simulink model "simulink_10_04_procede"  (R2024a)
settings: Solver=VariableStepAuto  StartTime=0.0  StopTime=600  RelTol=1e-3
StartFcn:
  | out = [];
  | disp(Consigne)
  |             disp(T_init);
  |             if Consigne > T_init
  |                 if T_init < 23
  |                     K1 = 0.007628;
  |                     T1 = 0.01103;
  |                     K2 = 0.03405;
  |                     T2 = 0.03035;
  |                     K3 = 0.04391;
  |                     T3 = 0.04924;
  |                 else
  |                     K1 = 0.00881;
  |                     T1 = 0.01194;
  |                     K2 = 0.02418;
  |                     T2 = 0.02359;
  |                     K3 = 0.04385;
  |                     T3 = 0.04942;
  |                 end
  |             else
  |                 if T_init < 30
  |                     K1 = 0.00751;
  |                     T1 = 0.01415;
  |                     K2 = 0.02291;
  |                     T2 = 0.02201;
  |                     K3 = 0.3512;
  |                     T3 = 0.3473;
  |                 else
  |                     K1 = 0.01043;
  |                     T1 = 0.01371;
  |                     K2 = 0.02568;
  |                     T2 = 0.0256;
  |                     K3 = 0.03719;
  |                     T3 = 0.04271;
  |                 end
  |             end
  |             disp('K1');
  |             disp(K1);
StopFcn:
  | try
  |     enreg = get_param('simulink_08_04_procede/Boucle Fermée', 'Enregistrement');
  |     nom = get_param('simulink_08_04_procede/Boucle Fermée', 'Fichier');
  | 
  |     if strcmp(enreg, 'on')
  |         dossier = fileparts(get_param('simulink_08_04_procede', 'FileName'));
  | 
  |         t = out.tout;
  |         y = out.Fichier;
  | 
  |         n = min(length(t), length(y));
  |         t_cut = t(1:n);
  |         y_cut = y(1:n, :);
  | 
  |         T = table(t_cut, y_cut(:,1), 'VariableNames', {'temps', 'sortie'});
  |         writetable(T, fullfile(dossier, [nom '.csv']));
  |     end
  | catch e
  |     disp(['Erreur exportation: ' e.message]);
  | end
values from neighbouring files (symbols this model uses):
  Consigne = ws.get('Consigne')    [logique.m]    (also in variables_simulation.m = 30)
  t_pertub_1 = 30    [variables_simulation.m]
  t_pertub_2 = 30    [variables_simulation.m]
  t_pertub_3 = 30    [variables_simulation.m]
settings Model: Creator=sabri  LastModifiedBy=MADER143
settings DataIOCC: OutputSaveName=y3

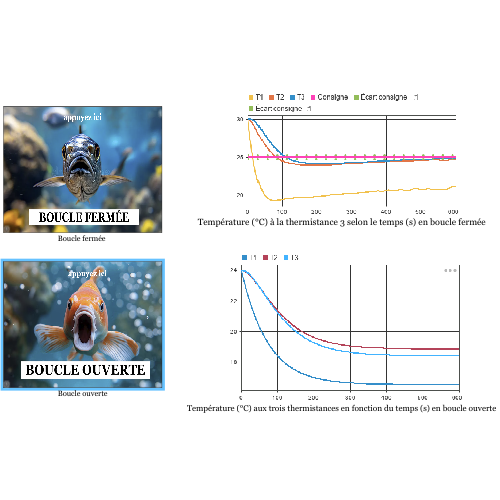
[thumbnail: Simulink's stored preview of the top-level diagram]
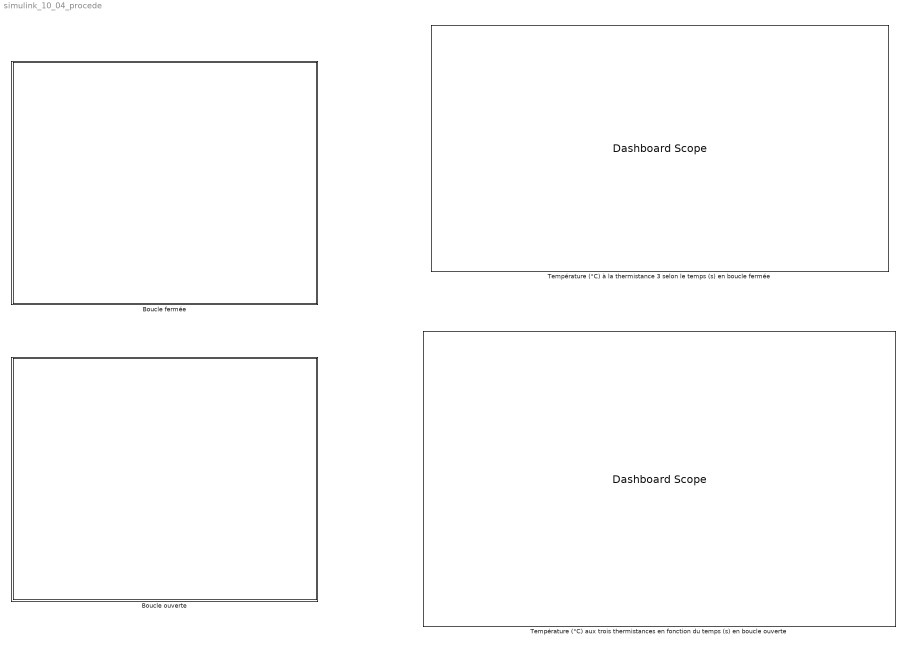
== system simulink_10_04_procede ==
  "Boucle fermée " : Subsystem  mask{Consigne=25, T_init=30, Temps=600, Enregistrement=on, Fichier=simulation, V1_3=1.79, Rg_3=5600, R1_3=3300, Rf_3=6300, B3=3700, V2_3=5, V1_2=1.8, Rg_2=5600, R1_2=3300, Rf_2=6300, B2=3984, V2_2=5, V1_1=1.774, Rg_1=5600, R1_1=3300, Rf_1=3300, B1=4010, V2_1=5, T_0=298.15, RT_0=10000, bz=-0.9726, az=0.0133, K1=0, T1=0, K2=0, T2=0, K3=0, T3=0, nb_bits=10, Ts=0.5, R=25, t_perturb_3=0, t_perturb_2=110, t_perturb_1=0, perturb_3=0, perturb_2=0.5, perturb_1=0, K=10.5, Ti=230, Td=40, PWM=0}
      mask prompts: Consigne "Température désirée"; T_init "Température initiale"; Temps "Durée de la simulation (s)"; Enregistrement "Enregistrer les données"; Fichier "Nom du fichier à enregistré:"; V1_3 "Tension d'alimentation de la branche positive de l'ampli-op (V)"; Rg_3 "Résistance en parallèle avec la thermitance (Ω)"; R1_3 "Résistance de la branche négative de l'ampli-op (Ω)"; Rf_3 "Résistance du trimpot (Ω)"; B3 "B"; V2_3 "Tension d'alimentation (V)"; V1_2 "Tension d'alimentation de la branche positive de l'ampli-op (V) de T1"; Rg_2 "Résistance en parallèle avec la thermitance (Ω)"; R1_2 "Résistance de la branche négative de l'ampli-op (Ω)"; Rf_2 "Résistance du trimpot (Ω)"; B2 "B"; V2_2 "Tension d'alimentation (V) de T1"; V1_1 "Tension d'alimentation de la branche positive de l'ampli-op (V) de T1"; Rg_1 "Résistance en parallèle avec la thermitance (Ω)"; R1_1 "Résistance de la branche négative de l'ampli-op (Ω)"; Rf_1 "Résistance du trimpot (Ω)"; B1 "B"; V2_1 "Tension d'alimentation (V) de T1"; T_0 "Température de référence de la thermistance (K)"; RT_0 "Résistance de référence de la thermistance (Ω)"; bz "Constante b"; az "Constante a"; K1 "Gain"; T1 "Constante de temps"; K2 "Gain"; T2 "Constante de temps"; K3 "Gain"; T3 "Constante de temps"; nb_bits "Nombre de bits du MC"; Ts "Fréquence d'échantillonnage"; R "Résistance de la perturbation (Ω)"; t_perturb_3 "Temps de la perturbation 3"; t_perturb_2 "Temps de la perturbation 2"; t_perturb_1 "Temps de la perturbation 1"; perturb_3 "Puissance de la perturbation à T3"; perturb_2 "Puissance de la perturbation à T2"; perturb_1 "Puissance de la perturbation à T1"; K "Gain"; Ti "Constante de temps intégrale"; Td "Constante de temps dérivée"
      mask DialogControl ParameterGroupVar Prompt: Simulateur
      mask DialogControl Container3 Prompt: Guide d'utilisation
      mask DialogControl Control2 Prompt: Voici le simulateur thermique de l'équipe 5. Vous pouvez modifier les valeurs des différents paramètres du prototype ci-dessus et choisir la température désirée.
      mask DialogControl Control3 Prompt: Lancer la simulation!
      mask DialogControl Container4 Prompt: Paramètres du prototype
      mask DialogControl Container8 Prompt: Paramètres des thermistances
      mask DialogControl Container9 Prompt: Thermistance 3
      mask DialogControl Container7 Prompt: Thermistance 2
      mask DialogControl Container5 Prompt: Thermistance 1
      mask DialogControl Container11 Prompt: Fonctions de transfert des thermistances
      mask DialogControl Container15 Prompt: T2 -> T3
      mask DialogControl Container12 Prompt: U -> V1
      mask DialogControl Container13 Prompt: V1 -> V2
      mask DialogControl Container14 Prompt: V2 -> V3
      mask DialogControl Container10 Prompt: Paramètres des perturbations
      mask DialogControl Container6 Prompt: Paramètres PID
      mask Display: image('boucle_fermee.png');
  Boucle ouverte : Subsystem  mask{PWM=-20, T_init=24, Temps=600, Enregistrement=on, Fichier=simulation, V1_3=1.79, Rg_3=5600, R1_3=3300, Rf_3=6300, B3=3700, V2_3=5, V1_2=1.8, Rg_2=5600, R1_2=3300, Rf_2=6300, B2=3984, V2_2=5, V1_1=1.774, Rg_1=5600, R1_1=3300, Rf_1=3300, B1=4010, V2_1=5, T_0=298.15, RT_0=10000, bz=-0.9726, az=0.0133, K1=0, T1=0, K2=0, T2=0, K3=0, T3=0, nb_bits=10, Ts=0.5, R=25, t_perturb_3=250, t_perturb_2=0, t_perturb_1=0, perturb_3=0, perturb_2=0, perturb_1=0, K=10.5, Ti=230, Td=40}
      mask prompts: PWM "PWM à envoyer"; T_init "Température initiale"; Temps "Durée de la simulation (s)"; Enregistrement "Enregistrer les données"; Fichier "Nom du fichier à enregistré:"; V1_3 "Tension d'alimentation de la branche positive de l'ampli-op (V)"; Rg_3 "Résistance en parallèle avec la thermitance (Ω)"; R1_3 "Résistance de la branche négative de l'ampli-op (Ω)"; Rf_3 "Résistance du trimpot (Ω)"; B3 "B"; V2_3 "Tension d'alimentation (V)"; V1_2 "Tension d'alimentation de la branche positive de l'ampli-op (V) de T1"; Rg_2 "Résistance en parallèle avec la thermitance (Ω)"; R1_2 "Résistance de la branche négative de l'ampli-op (Ω)"; Rf_2 "Résistance du trimpot (Ω)"; B2 "B"; V2_2 "Tension d'alimentation (V) de T1"; V1_1 "Tension d'alimentation de la branche positive de l'ampli-op (V) de T1"; Rg_1 "Résistance en parallèle avec la thermitance (Ω)"; R1_1 "Résistance de la branche négative de l'ampli-op (Ω)"; Rf_1 "Résistance du trimpot (Ω)"; B1 "B"; V2_1 "Tension d'alimentation (V) de T1"; T_0 "Température de référence de la thermistance (K)"; RT_0 "Résistance de référence de la thermistance (Ω)"; bz "Constante b"; az "Constante a"; K1 "Gain"; T1 "Constante de temps"; K2 "Gain"; T2 "Constante de temps"; K3 "Gain"; T3 "Constante de temps"; nb_bits "Nombre de bits du MC"; Ts "Fréquence d'échantillonnage"; R "Résistance de la perturbation (Ω)"; t_perturb_3 "Temps de la perturbation 3"; t_perturb_2 "Temps de la perturbation 2"; t_perturb_1 "Temps de la perturbation 1"; perturb_3 "Puissance de la perturbation à T3"; perturb_2 "Puissance de la perturbation à T2"; perturb_1 "Puissance de la perturbation à T1"; K "Gain"; Ti "Constante de temps intégrale"; Td "Constante de temps dérivée"
      mask DialogControl ParameterGroupVar Prompt: Simulateur
      mask DialogControl Container3 Prompt: Guide d'utilisation
      mask DialogControl Control2 Prompt: Voici le simulateur thermique en boucle ouverte de l'équipe 5. Vous pouvez modifier les valeurs des différents paramètres du prototype ci-dessus et choisir la consigne en PWM.
      mask DialogControl Control3 Prompt: Lancer la simulation!
      mask DialogControl Container4 Prompt: Paramètres du prototype
      mask DialogControl Container8 Prompt: Paramètres des thermistances
      mask DialogControl Container9 Prompt: Thermistance 3
      mask DialogControl Container7 Prompt: Thermistance 2
      mask DialogControl Container5 Prompt: Thermistance 1
      mask DialogControl Container11 Prompt: Fonctions de transfert des thermistances
      mask DialogControl Container15 Prompt: T2 -> T3
      mask DialogControl Container12 Prompt: U -> V1
      mask DialogControl Container13 Prompt: V1 -> V2
      mask DialogControl Container14 Prompt: V2 -> V3
      mask DialogControl Container10 Prompt: Paramètres des perturbations
      mask DialogControl Container6 Prompt: Paramètres PID
      mask Display: image('boucle_ouverte.png');
  Température (°C) aux trois thermistances en fonction du temps (s) en boucle ouverte : DashboardScope
  Température (°C) à la thermistance 3 selon le temps (s) en boucle fermée : DashboardScope

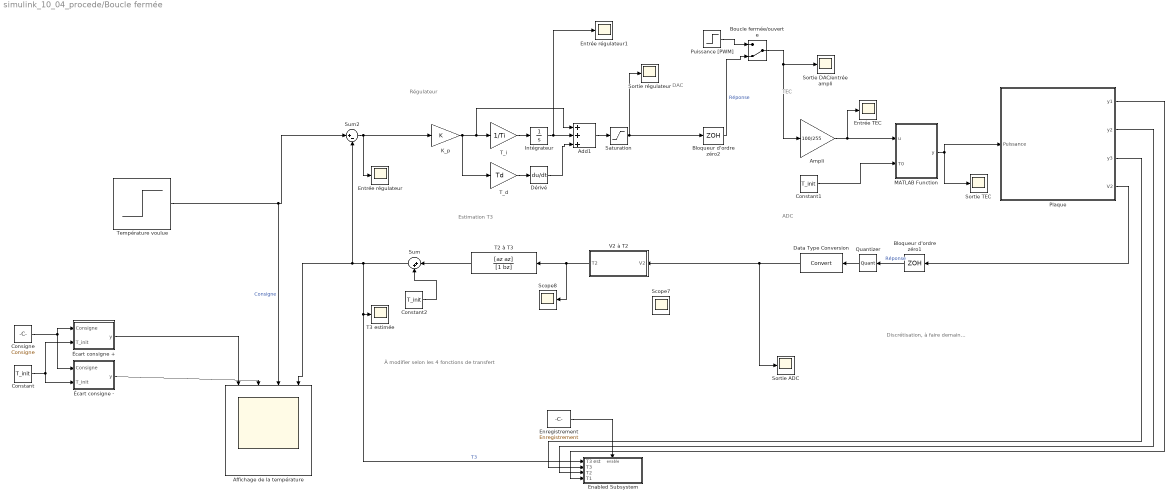
== system simulink_10_04_procede/Boucle fermée  ==
  note: À modifier selon les 4 fonctions de transfert
  note: Discrétisation, à faire demain...
  note: TEC
  note: DAC
  note: Régulateur
  note: Estimation T3
  note: ADC
  Add1 : Sum  Inputs=+++
  Affichage de la température : Scope  NumInputPorts=4
  Ampli : Gain  Gain=100/255
  Bloqueur d'ordre zéro1 : ZeroOrderHold  SampleTime=Ts
  Bloqueur d'ordre zéro2 : ZeroOrderHold  SampleTime=Ts
  Boucle fermée/ouverte : ManualSwitch  CurrentSetting=0
  Consigne : Constant  Value=Consigne
  Constant : Constant  Value=T_init
  Constant1 : Constant  Value=T_init
  Constant2 : Constant  Value=T_init
  Data Type Conversion : DataTypeConversion  OutMin=[-5]  OutMax=[5]  SaturateOnIntegerOverflow=off  RndMeth=Floor
  Dérivé : Derivative
  Enabled Subsystem : Subsystem  TreatAsAtomicUnit=on
  Enregistrement : Constant  Value=Enregistrement
  Entrée TEC : Scope
  Entrée régulateur : Scope
  Entrée régulateur1 : Scope
  Intégrateur : Integrator
  K_p : Gain  Gain=K
  MATLAB Function : MATLAB Function  TreatAsAtomicUnit=on
  Plaque : Subsystem
  Puissance [PWM] : Step  After=20  SampleTime=0
  Quantizer : Quantizer  QuantizationInterval=nb_bits/1023
  Saturation : Saturate  UpperLimit=70  LowerLimit=-70
  Scope7 : Scope
  Scope8 : Scope
  Sortie ADC : Scope
  Sortie DAC/entrée ampli : Scope
  Sortie TEC : Scope
  Sortie régulateur : Scope
  Sum : Sum  Inputs=|++
  Sum2 : Sum  Inputs=|+-
  T2 à T3 : DiscreteTransferFcn  Numerator=[az az]  Denominator=[1 bz]
  T3 estimée : Scope
  T_d : Gain  Gain=Td
  T_i : Gain  Gain=1/Ti
  Température voulue : Step  Time=0  Before=T_init  After=Consigne  SampleTime=0
  V2 à T2 : Subsystem
  Écart consigne + : MATLAB Function  TreatAsAtomicUnit=on
  Écart consigne - : MATLAB Function  TreatAsAtomicUnit=on
  wires:
  Écart consigne -/1(y) -> Affichage de la température/2
  Température voulue/1 -> Sum2/1, Affichage de la température/3  "Consigne"
  Écart consigne +/1(y) -> Affichage de la température/1
  Enregistrement/1 -> Enabled Subsystem/Enable
  Consigne/1 -> Écart consigne -/1(Consigne), Écart consigne +/1(Consigne)
  Constant/1 -> Écart consigne -/2(T_init), Écart consigne +/2(T_init)
  Boucle fermée/ouverte/1 -> Ampli/1, Sortie DAC/entrée ampli/1
  Intégrateur/1 -> Entrée régulateur1/1, Add1/2
  MATLAB Function/1(y) -> Plaque/1(Puissance), Sortie TEC/1
  Puissance [PWM]/1 -> Boucle fermée/ouverte/1
  Constant1/1 -> MATLAB Function/2(T0)
  Ampli/1 -> Entrée TEC/1, MATLAB Function/1(u)
  Sum2/1 -> Entrée régulateur/1, K_p/1
  T_i/1 -> Intégrateur/1
  Constant2/1 -> Sum/2
  V2 à T2/1(T2) -> T2 à T3/1, Scope8/1
  T2 à T3/1 -> Sum/1
  Add1/1 -> Saturation/1
  Saturation/1 -> Bloqueur d'ordre zéro2/1, Sortie régulateur/1
  Sum/1 -> Enabled Subsystem/1(T3 est), T3 estimée/1, Affichage de la température/4, Sum2/2  "T3"
  Quantizer/1 -> Data Type Conversion/1
  Plaque/4(V2) -> Bloqueur d'ordre zéro1/1
  Bloqueur d'ordre zéro1/1 -> Quantizer/1  "Réponse"
  Data Type Conversion/1 -> Sortie ADC/1, V2 à T2/1(V2)
  Bloqueur d'ordre zéro2/1 -> Boucle fermée/ouverte/2  "Réponse"
  K_p/1 -> T_d/1, Add1/1, T_i/1
  Dérivé/1 -> Add1/3
  T_d/1 -> Dérivé/1
  Plaque/2(y2) -> Enabled Subsystem/3(T2)
  Plaque/3(y3) -> Enabled Subsystem/2(T3)
  Plaque/1(y1) -> Enabled Subsystem/4(T1)

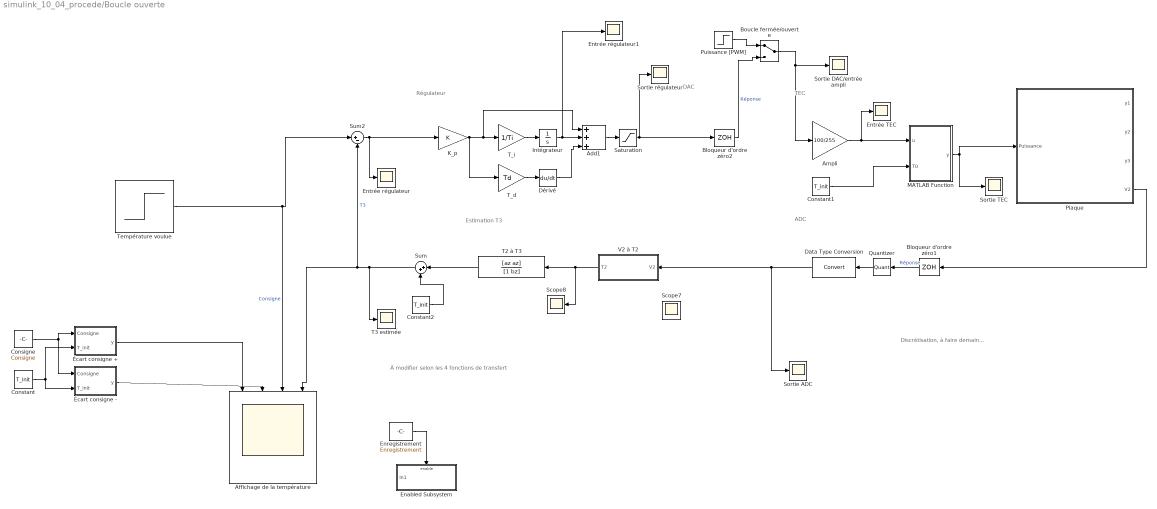
== system simulink_10_04_procede/Boucle ouverte ==
  note: À modifier selon les 4 fonctions de transfert
  note: Discrétisation, à faire demain...
  note: TEC
  note: DAC
  note: Régulateur
  note: Estimation T3
  note: ADC
  Add1 : Sum  Inputs=+++
  Affichage de la température : Scope  NumInputPorts=4
  Ampli : Gain  Gain=100/255
  Bloqueur d'ordre zéro1 : ZeroOrderHold  SampleTime=Ts
  Bloqueur d'ordre zéro2 : ZeroOrderHold  SampleTime=Ts
  Boucle fermée/ouverte : ManualSwitch
  Consigne : Constant  Value=Consigne
  Constant : Constant  Value=T_init
  Constant1 : Constant  Value=T_init
  Constant2 : Constant  Value=T_init
  Data Type Conversion : DataTypeConversion  OutMin=[-5]  OutMax=[5]  SaturateOnIntegerOverflow=off  RndMeth=Floor
  Dérivé : Derivative
  Enabled Subsystem : Subsystem  TreatAsAtomicUnit=on
  Enregistrement : Constant  Value=Enregistrement
  Entrée TEC : Scope
  Entrée régulateur : Scope
  Entrée régulateur1 : Scope
  Intégrateur : Integrator
  K_p : Gain  Gain=K
  MATLAB Function : MATLAB Function  TreatAsAtomicUnit=on
  Plaque : Subsystem
  Puissance [PWM] : Step  After=PWM  SampleTime=0
  Quantizer : Quantizer  QuantizationInterval=nb_bits/1023
  Saturation : Saturate  UpperLimit=70  LowerLimit=-70
  Scope7 : Scope
  Scope8 : Scope
  Sortie ADC : Scope
  Sortie DAC/entrée ampli : Scope
  Sortie TEC : Scope
  Sortie régulateur : Scope
  Sum : Sum  Inputs=|++
  Sum2 : Sum  Inputs=|+-
  T2 à T3 : DiscreteTransferFcn  Numerator=[az az]  Denominator=[1 bz]
  T3 estimée : Scope
  T_d : Gain  Gain=Td
  T_i : Gain  Gain=1/Ti
  Température voulue : Step  Time=0  Before=T_init  After=Consigne  SampleTime=0
  V2 à T2 : Subsystem
  Écart consigne + : MATLAB Function  TreatAsAtomicUnit=on
  Écart consigne - : MATLAB Function  TreatAsAtomicUnit=on
  wires:
  Écart consigne -/1(y) -> Affichage de la température/2
  Température voulue/1 -> Sum2/1, Affichage de la température/3  "Consigne"
  Écart consigne +/1(y) -> Affichage de la température/1
  Enregistrement/1 -> Enabled Subsystem/Enable
  Consigne/1 -> Écart consigne -/1(Consigne), Écart consigne +/1(Consigne)
  Constant/1 -> Écart consigne -/2(T_init), Écart consigne +/2(T_init)
  Boucle fermée/ouverte/1 -> Ampli/1, Sortie DAC/entrée ampli/1
  Intégrateur/1 -> Entrée régulateur1/1, Add1/2
  MATLAB Function/1(y) -> Plaque/1(Puissance), Sortie TEC/1
  Puissance [PWM]/1 -> Boucle fermée/ouverte/1
  Constant1/1 -> MATLAB Function/2(T0)
  Ampli/1 -> Entrée TEC/1, MATLAB Function/1(u)
  Sum2/1 -> Entrée régulateur/1, K_p/1
  T_i/1 -> Intégrateur/1
  Constant2/1 -> Sum/2
  V2 à T2/1(T2) -> T2 à T3/1, Scope8/1
  T2 à T3/1 -> Sum/1
  Add1/1 -> Saturation/1
  Saturation/1 -> Bloqueur d'ordre zéro2/1, Sortie régulateur/1
  Sum/1 -> T3 estimée/1, Affichage de la température/4, Sum2/2  "T3"
  Quantizer/1 -> Data Type Conversion/1
  Plaque/4(V2) -> Bloqueur d'ordre zéro1/1
  Bloqueur d'ordre zéro1/1 -> Quantizer/1  "Réponse"
  Data Type Conversion/1 -> Sortie ADC/1, V2 à T2/1(V2)
  Bloqueur d'ordre zéro2/1 -> Boucle fermée/ouverte/2  "Réponse"
  K_p/1 -> T_d/1, Add1/1, T_i/1
  Dérivé/1 -> Add1/3
  T_d/1 -> Dérivé/1

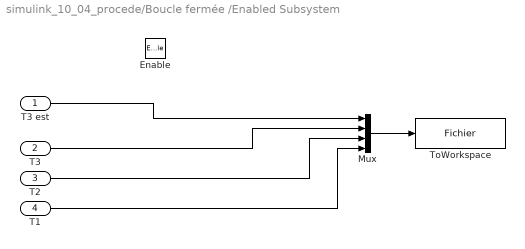
== system simulink_10_04_procede/Boucle fermée /Enabled Subsystem ==
  T3 est : Inport
  T3 : Inport  Port=2
  T2 : Inport  Port=3
  T1 : Inport  Port=4
  Enable : EnablePort
  Mux : Mux
  ToWorkspace : ToWorkspace  VariableName=Fichier  SaveFormat=Timeseries  SampleTime=0.5
  wires:
  T3/1 -> Mux/2
  Mux/1 -> ToWorkspace/1
  T3 est/1 -> Mux/1
  T2/1 -> Mux/3
  T1/1 -> Mux/4

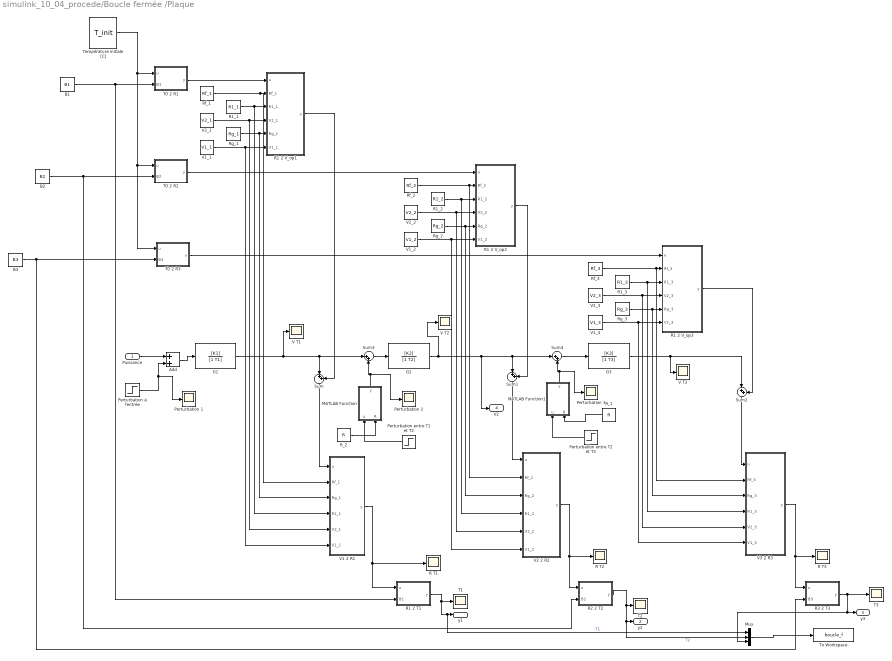
== system simulink_10_04_procede/Boucle fermée /Plaque ==
  Puissance : Inport
  Add : Sum
  B1 : Constant  Value=B1
  B2 : Constant  Value=B2
  B3 : Constant  Value=B3
  G1 : TransferFcn  Numerator=[K1]  Denominator=[1 T1]
  G2 : TransferFcn  Numerator=[K2]  Denominator=[1 T2]
  G3 : TransferFcn  Numerator=[K3]  Denominator=[1 T3]
  MATLAB Function : MATLAB Function  TreatAsAtomicUnit=on
  MATLAB Function1 : MATLAB Function  TreatAsAtomicUnit=on
  Mux : Mux  Inputs=3
  Perturbation 1 : Scope
  Perturbation 2 : Scope
  Perturbation 3 : Scope
  Perturbation entre T1 et T2 : Step  Time=t_pertub_2  After=perturb_2  SampleTime=0
  Perturbation entre T2 et T3 : Step  Time=t_pertub_3  After=perturb_3  SampleTime=0
  Perturbation à l'entrée : Step  Time=t_pertub_1  After=perturb_1  SampleTime=0
  R T1 : Scope
  R T2 : Scope
  R T3 : Scope
  R1 2 T1 : MATLAB Function  TreatAsAtomicUnit=on
  R1 2 V_op1 : MATLAB Function  TreatAsAtomicUnit=on
  R1 2 V_op2 : MATLAB Function  TreatAsAtomicUnit=on
  R1 2 V_op3 : MATLAB Function  TreatAsAtomicUnit=on
  R1_1 : Constant  Value=R1_1
  R1_2 : Constant  Value=R1_2
  R1_3 : Constant  Value=R1_3
  R2 2 T2 : MATLAB Function  TreatAsAtomicUnit=on
  R3 2 T3 : MATLAB Function  TreatAsAtomicUnit=on
  R_1 : Constant  Value=R
  R_2 : Constant  Value=R
  Rf_1 : Constant  Value=Rf_1
  Rf_2 : Constant  Value=Rf_2
  Rf_3 : Constant  Value=Rf_3
  Rg_1 : Constant  Value=Rg_1
  Rg_2 : Constant  Value=Rg_2
  Rg_3 : Constant  Value=Rg_3
  Sum{,1..4} (5 alike) : Sum  Inputs=|++
  T0 2 R1 : MATLAB Function  TreatAsAtomicUnit=on
  T0 2 R2 : MATLAB Function  TreatAsAtomicUnit=on
  T0 2 R3 : MATLAB Function  TreatAsAtomicUnit=on
  T1 : Scope
  T2 : Scope
  T3 : Scope
  Température initiale [C] : Constant  Value=T_init
  To Workspace : ToWorkspace  VariableName=boucle_f  SaveFormat=Timeseries  SampleTime=-1
  V T1 : Scope
  V T2 : Scope
  V T3 : Scope
  V1 2 R1 : MATLAB Function  TreatAsAtomicUnit=on
  V1_1 : Constant  Value=V1_1
  V1_2 : Constant  Value=V1_2
  V1_3 : Constant  Value=V1_3
  V2 2 R2 : MATLAB Function  TreatAsAtomicUnit=on
  V2_1 : Constant  Value=V2_1
  V2_2 : Constant  Value=V2_2
  V2_3 : Constant  Value=V2_3
  V3 2 R3 : MATLAB Function  TreatAsAtomicUnit=on
  y1 : Outport
  y2 : Outport  Port=2
  y3 : Outport  Port=3
  V2 : Outport  Port=4
  wires:
  G2/1 -> V T2/1, V2/1, Sum1/1, Sum4/1
  R3 2 T3/1(y) -> Mux/3, y3/1, T3/1
  V1 2 R1/1(y) -> R T1/1, R1 2 T1/1(u)
  G3/1 -> V T3/1, Sum2/1
  T0 2 R3/1(y) -> R1 2 V_op3/1(u)
  Sum/1 -> V1 2 R1/1(u)
  R1 2 V_op1/1(y) -> Sum/2
  Add/1 -> G1/1
  T0 2 R2/1(y) -> R1 2 V_op2/1(u)
  R1 2 V_op3/1(y) -> Sum2/2
  R1 2 V_op2/1(y) -> Sum1/2
  Sum2/1 -> V3 2 R3/1(u)
  T0 2 R1/1(y) -> R1 2 V_op1/1(u)
  R1 2 T1/1(y) -> Mux/1, y1/1, T1/1  "T1"
  Sum1/1 -> V2 2 R2/1(u)
  Température initiale [C]/1 -> T0 2 R3/1(u), T0 2 R2/1(u), T0 2 R1/1(u)
  G1/1 -> Sum3/1, Sum/1, V T1/1
  Perturbation à l'entrée/1 -> Perturbation 1/1, Add/2
  B2/1 -> T0 2 R2/2(B2), R2 2 T2/2(B2)
  B3/1 -> R3 2 T3/2(B3), T0 2 R3/2(B3)
  Puissance/1 -> Add/1
  Sum3/1 -> G2/1
  Sum4/1 -> G3/1
  V2 2 R2/1(y) -> R T2/1, R2 2 T2/1(u)
  B1/1 -> R1 2 T1/2(B1), T0 2 R1/2(B1)
  R2 2 T2/1(y) -> Mux/2, y2/1, T2/1  "T2"
  Rf_1/1 -> V1 2 R1/2(Rf_1), R1 2 V_op1/2(Rf_1)
  R1_1/1 -> V1 2 R1/4(R1_1), R1 2 V_op1/3(R1_1)
  V2_1/1 -> R1 2 V_op1/4(V2_1), V1 2 R1/5(V2_1)
  Rg_1/1 -> R1 2 V_op1/5(Rg_1), V1 2 R1/3(Rg_1)
  V1_1/1 -> V1 2 R1/6(V1_1), R1 2 V_op1/6(V1_1)
  Rf_2/1 -> V2 2 R2/2(Rf_2), R1 2 V_op2/2(Rf_2)
  R1_2/1 -> V2 2 R2/4(R1_2), R1 2 V_op2/3(R1_2)
  V2_2/1 -> V2 2 R2/5(V2_2), R1 2 V_op2/4(V2_2)
  Rg_2/1 -> V2 2 R2/3(Rg_2), R1 2 V_op2/5(Rg_2)
  V1_2/1 -> V2 2 R2/6(V1_2), R1 2 V_op2/6(V1_2)
  Rf_3/1 -> V3 2 R3/2(Rf_3), R1 2 V_op3/2(Rf_3)
  R1_3/1 -> V3 2 R3/4(R1_3), R1 2 V_op3/3(R1_3)
  V2_3/1 -> V3 2 R3/5(V2_3), R1 2 V_op3/4(V2_3)
  Rg_3/1 -> V3 2 R3/3(Rg_3), R1 2 V_op3/5(Rg_3)
  V1_3/1 -> V3 2 R3/6(V1_3), R1 2 V_op3/6(V1_3)
  V3 2 R3/1(y) -> R T3/1, R3 2 T3/1(u)
  Mux/1 -> To Workspace/1
  MATLAB Function/1(y) -> Sum3/2, Perturbation 2/1
  Perturbation entre T1 et T2/1 -> MATLAB Function/1(u)
  MATLAB Function1/1(y) -> Sum4/2, Perturbation 3/1
  Perturbation entre T2 et T3/1 -> MATLAB Function1/1(u)
  R_2/1 -> MATLAB Function/2(R)
  R_1/1 -> MATLAB Function1/2(R)

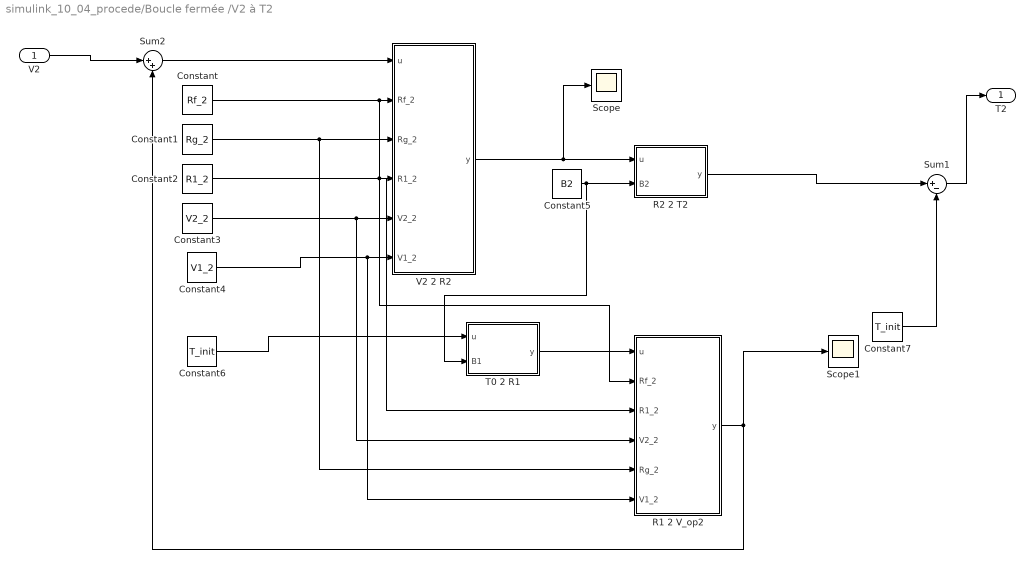
== system simulink_10_04_procede/Boucle fermée /V2 à T2 ==
  V2 : Inport
  Constant : Constant  Value=Rf_2
  Constant1 : Constant  Value=Rg_2
  Constant2 : Constant  Value=R1_2
  Constant3 : Constant  Value=V2_2
  Constant4 : Constant  Value=V1_2
  Constant5 : Constant  Value=B2
  Constant6 : Constant  Value=T_init
  Constant7 : Constant  Value=T_init
  R1 2 V_op2 : MATLAB Function  TreatAsAtomicUnit=on
  R2 2 T2 : MATLAB Function  TreatAsAtomicUnit=on
  Scope : Scope
  Scope1 : Scope
  Sum1 : Sum  Inputs=|+-
  Sum2 : Sum  Inputs=|++
  T0 2 R1 : MATLAB Function  TreatAsAtomicUnit=on
  V2 2 R2 : MATLAB Function  TreatAsAtomicUnit=on
  T2 : Outport
  wires:
  Constant/1 -> R1 2 V_op2/2(Rf_2), V2 2 R2/2(Rf_2)
  Constant1/1 -> R1 2 V_op2/5(Rg_2), V2 2 R2/3(Rg_2)
  Constant2/1 -> R1 2 V_op2/3(R1_2), V2 2 R2/4(R1_2)
  Constant3/1 -> V2 2 R2/5(V2_2), R1 2 V_op2/4(V2_2)
  Constant4/1 -> V2 2 R2/6(V1_2), R1 2 V_op2/6(V1_2)
  Constant5/1 -> T0 2 R1/2(B1), R2 2 T2/2(B2)
  T0 2 R1/1(y) -> R1 2 V_op2/1(u)
  Constant6/1 -> T0 2 R1/1(u)
  R1 2 V_op2/1(y) -> Scope1/1, Sum2/2
  V2 2 R2/1(y) -> Scope/1, R2 2 T2/1(u)
  R2 2 T2/1(y) -> Sum1/1
  Sum1/1 -> T2/1
  Constant7/1 -> Sum1/2
  V2/1 -> Sum2/1
  Sum2/1 -> V2 2 R2/1(u)

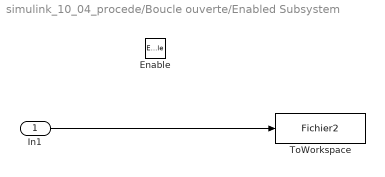
== system simulink_10_04_procede/Boucle ouverte/Enabled Subsystem ==
  In1 : Inport
  Enable : EnablePort
  ToWorkspace : ToWorkspace  VariableName=Fichier2  SampleTime=0.5
  wires:
  In1/1 -> ToWorkspace/1

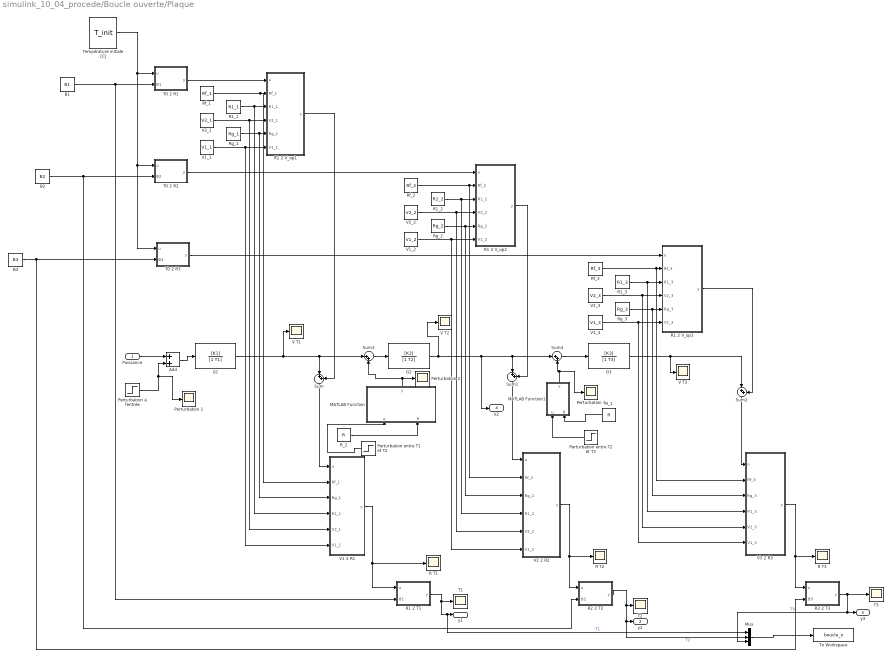
== system simulink_10_04_procede/Boucle ouverte/Plaque ==
  Puissance : Inport
  Add : Sum
  B1 : Constant  Value=B1
  B2 : Constant  Value=B2
  B3 : Constant  Value=B3
  G1 : TransferFcn  Numerator=[K1]  Denominator=[1 T1]
  G2 : TransferFcn  Numerator=[K2]  Denominator=[1 T2]
  G3 : TransferFcn  Numerator=[K3]  Denominator=[1 T3]
  MATLAB Function : MATLAB Function  TreatAsAtomicUnit=on
  MATLAB Function1 : MATLAB Function  TreatAsAtomicUnit=on
  Mux : Mux  Inputs=3
  Perturbation 1 : Scope
  Perturbation 2 : Scope
  Perturbation 3 : Scope
  Perturbation entre T1 et T2 : Step  Time=t_pertub_2  After=perturb_2  SampleTime=0
  Perturbation entre T2 et T3 : Step  Time=t_pertub_3  After=perturb_3  SampleTime=0
  Perturbation à l'entrée : Step  Time=t_pertub_1  After=perturb_1  SampleTime=0
  R T1 : Scope
  R T2 : Scope
  R T3 : Scope
  R1 2 T1 : MATLAB Function  TreatAsAtomicUnit=on
  R1 2 V_op1 : MATLAB Function  TreatAsAtomicUnit=on
  R1 2 V_op2 : MATLAB Function  TreatAsAtomicUnit=on
  R1 2 V_op3 : MATLAB Function  TreatAsAtomicUnit=on
  R1_1 : Constant  Value=R1_1
  R1_2 : Constant  Value=R1_2
  R1_3 : Constant  Value=R1_3
  R2 2 T2 : MATLAB Function  TreatAsAtomicUnit=on
  R3 2 T3 : MATLAB Function  TreatAsAtomicUnit=on
  R_1 : Constant  Value=R
  R_2 : Constant  Value=R
  Rf_1 : Constant  Value=Rf_1
  Rf_2 : Constant  Value=Rf_2
  Rf_3 : Constant  Value=Rf_3
  Rg_1 : Constant  Value=Rg_1
  Rg_2 : Constant  Value=Rg_2
  Rg_3 : Constant  Value=Rg_3
  Sum{,1..4} (5 alike) : Sum  Inputs=|++
  T0 2 R1 : MATLAB Function  TreatAsAtomicUnit=on
  T0 2 R2 : MATLAB Function  TreatAsAtomicUnit=on
  T0 2 R3 : MATLAB Function  TreatAsAtomicUnit=on
  T1 : Scope
  T2 : Scope
  T3 : Scope
  Température initiale [C] : Constant  Value=T_init
  To Workspace : ToWorkspace  VariableName=boucle_o  SaveFormat=Timeseries  SampleTime=-1
  V T1 : Scope
  V T2 : Scope
  V T3 : Scope
  V1 2 R1 : MATLAB Function  TreatAsAtomicUnit=on
  V1_1 : Constant  Value=V1_1
  V1_2 : Constant  Value=V1_2
  V1_3 : Constant  Value=V1_3
  V2 2 R2 : MATLAB Function  TreatAsAtomicUnit=on
  V2_1 : Constant  Value=V2_1
  V2_2 : Constant  Value=V2_2
  V2_3 : Constant  Value=V2_3
  V3 2 R3 : MATLAB Function  TreatAsAtomicUnit=on
  y1 : Outport
  y2 : Outport  Port=2
  y3 : Outport  Port=3
  V2 : Outport  Port=4
  wires:
  G2/1 -> V T2/1, V2/1, Sum1/1, Sum4/1
  R3 2 T3/1(y) -> Mux/3, y3/1, T3/1  "T3"
  V1 2 R1/1(y) -> R T1/1, R1 2 T1/1(u)
  G3/1 -> V T3/1, Sum2/1
  T0 2 R3/1(y) -> R1 2 V_op3/1(u)
  Sum/1 -> V1 2 R1/1(u)
  R1 2 V_op1/1(y) -> Sum/2
  Add/1 -> G1/1
  T0 2 R2/1(y) -> R1 2 V_op2/1(u)
  R1 2 V_op3/1(y) -> Sum2/2
  R1 2 V_op2/1(y) -> Sum1/2
  Sum2/1 -> V3 2 R3/1(u)
  T0 2 R1/1(y) -> R1 2 V_op1/1(u)
  R1 2 T1/1(y) -> Mux/1, y1/1, T1/1  "T1"
  Sum1/1 -> V2 2 R2/1(u)
  Température initiale [C]/1 -> T0 2 R3/1(u), T0 2 R2/1(u), T0 2 R1/1(u)
  G1/1 -> Sum3/1, Sum/1, V T1/1
  Perturbation à l'entrée/1 -> Perturbation 1/1, Add/2
  B2/1 -> T0 2 R2/2(B2), R2 2 T2/2(B2)
  B3/1 -> R3 2 T3/2(B3), T0 2 R3/2(B3)
  Puissance/1 -> Add/1
  Sum3/1 -> G2/1
  Sum4/1 -> G3/1
  V2 2 R2/1(y) -> R T2/1, R2 2 T2/1(u)
  B1/1 -> R1 2 T1/2(B1), T0 2 R1/2(B1)
  R2 2 T2/1(y) -> Mux/2, y2/1, T2/1  "T2"
  Rf_1/1 -> V1 2 R1/2(Rf_1), R1 2 V_op1/2(Rf_1)
  R1_1/1 -> V1 2 R1/4(R1_1), R1 2 V_op1/3(R1_1)
  V2_1/1 -> R1 2 V_op1/4(V2_1), V1 2 R1/5(V2_1)
  Rg_1/1 -> R1 2 V_op1/5(Rg_1), V1 2 R1/3(Rg_1)
  V1_1/1 -> V1 2 R1/6(V1_1), R1 2 V_op1/6(V1_1)
  Rf_2/1 -> V2 2 R2/2(Rf_2), R1 2 V_op2/2(Rf_2)
  R1_2/1 -> V2 2 R2/4(R1_2), R1 2 V_op2/3(R1_2)
  V2_2/1 -> V2 2 R2/5(V2_2), R1 2 V_op2/4(V2_2)
  Rg_2/1 -> V2 2 R2/3(Rg_2), R1 2 V_op2/5(Rg_2)
  V1_2/1 -> V2 2 R2/6(V1_2), R1 2 V_op2/6(V1_2)
  Rf_3/1 -> V3 2 R3/2(Rf_3), R1 2 V_op3/2(Rf_3)
  R1_3/1 -> V3 2 R3/4(R1_3), R1 2 V_op3/3(R1_3)
  V2_3/1 -> V3 2 R3/5(V2_3), R1 2 V_op3/4(V2_3)
  Rg_3/1 -> V3 2 R3/3(Rg_3), R1 2 V_op3/5(Rg_3)
  V1_3/1 -> V3 2 R3/6(V1_3), R1 2 V_op3/6(V1_3)
  V3 2 R3/1(y) -> R T3/1, R3 2 T3/1(u)
  Mux/1 -> To Workspace/1
  MATLAB Function/1(y) -> Sum3/2, Perturbation 2/1
  Perturbation entre T1 et T2/1 -> MATLAB Function/1(u)
  MATLAB Function1/1(y) -> Sum4/2, Perturbation 3/1
  Perturbation entre T2 et T3/1 -> MATLAB Function1/1(u)
  R_2/1 -> MATLAB Function/2(R)
  R_1/1 -> MATLAB Function1/2(R)

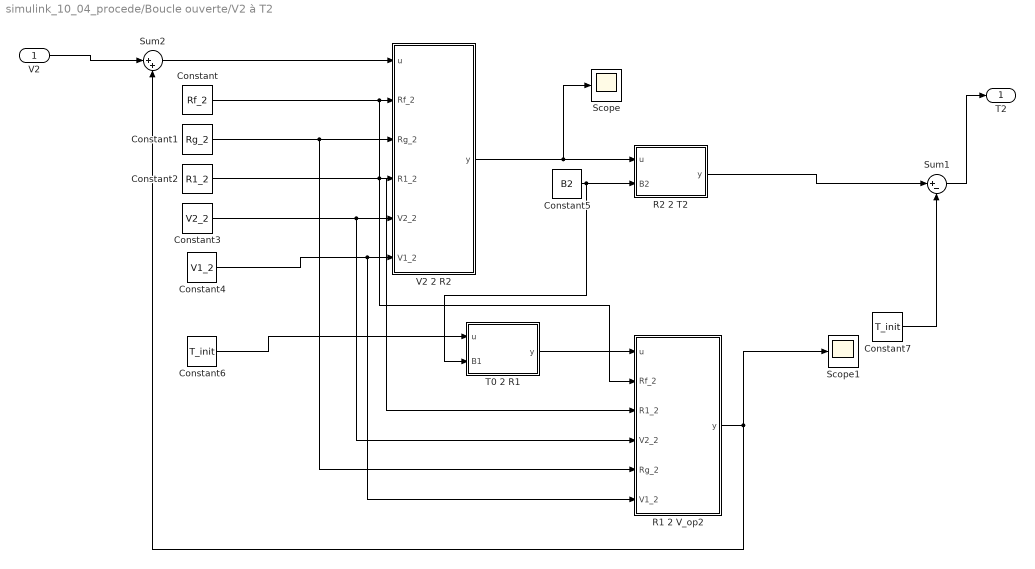
== system simulink_10_04_procede/Boucle ouverte/V2 à T2 ==
  V2 : Inport
  Constant : Constant  Value=Rf_2
  Constant1 : Constant  Value=Rg_2
  Constant2 : Constant  Value=R1_2
  Constant3 : Constant  Value=V2_2
  Constant4 : Constant  Value=V1_2
  Constant5 : Constant  Value=B2
  Constant6 : Constant  Value=T_init
  Constant7 : Constant  Value=T_init
  R1 2 V_op2 : MATLAB Function  TreatAsAtomicUnit=on
  R2 2 T2 : MATLAB Function  TreatAsAtomicUnit=on
  Scope : Scope
  Scope1 : Scope
  Sum1 : Sum  Inputs=|+-
  Sum2 : Sum  Inputs=|++
  T0 2 R1 : MATLAB Function  TreatAsAtomicUnit=on
  V2 2 R2 : MATLAB Function  TreatAsAtomicUnit=on
  T2 : Outport
  wires:
  Constant/1 -> R1 2 V_op2/2(Rf_2), V2 2 R2/2(Rf_2)
  Constant1/1 -> R1 2 V_op2/5(Rg_2), V2 2 R2/3(Rg_2)
  Constant2/1 -> R1 2 V_op2/3(R1_2), V2 2 R2/4(R1_2)
  Constant3/1 -> V2 2 R2/5(V2_2), R1 2 V_op2/4(V2_2)
  Constant4/1 -> V2 2 R2/6(V1_2), R1 2 V_op2/6(V1_2)
  Constant5/1 -> T0 2 R1/2(B1), R2 2 T2/2(B2)
  T0 2 R1/1(y) -> R1 2 V_op2/1(u)
  Constant6/1 -> T0 2 R1/1(u)
  R1 2 V_op2/1(y) -> Scope1/1, Sum2/2
  V2 2 R2/1(y) -> Scope/1, R2 2 T2/1(u)
  R2 2 T2/1(y) -> Sum1/1
  Sum1/1 -> T2/1
  Constant7/1 -> Sum1/2
  V2/1 -> Sum2/1
  Sum2/1 -> V2 2 R2/1(u)

== matlab function simulink_10_04_procede/Boucle fermée /Plaque/R1 2 T1 ==
  data: u input; y output; B1 input
function y = fcn(u, B1)
disp('B1');
disp(B1);
disp(u);
y = (1/((log(u/10000)/B1)+(1/(298.15))))-273.15;

== matlab function simulink_10_04_procede/Boucle fermée /Plaque/R2 2 T2 ==
  data: u input; y output; B2 input
function y = fcn(u, B2)
y = (1/((log(u/10000)/B2)+(1/(298.15))))-273.15;

== matlab function simulink_10_04_procede/Boucle fermée /Plaque/R3 2 T3 ==
  data: u input; y output; B3 input
function y = fcn(u, B3)

y = (1/((log(u/10000)/B3)+(1/(298.15))))-273.15;

== matlab function simulink_10_04_procede/Boucle fermée /Plaque/T0 2 R1 ==
  data: u input; y output; B1 input
function y = fcn(u, B1)
y = 10000*exp(B1*(1/(u+273.15) - 1/(298.15)));

== matlab function simulink_10_04_procede/Boucle fermée /Plaque/R1 2 V_op1 ==
  data: u input; y output; Rf_1 input; R1_1 input; V2_1 input; Rg_1 input; V1_1 input
function y = fcn_1(u, Rf_1, R1_1, V2_1, Rg_1, V1_1)

y = ((((Rf_1 + R1_1) * Rg_1 * V2_1) / (u + Rg_1)) - Rf_1 * V1_1) / R1_1;

== matlab function simulink_10_04_procede/Boucle fermée /Plaque/R1 2 V_op2 ==
  data: u input; y output; Rf_2 input; R1_2 input; V2_2 input; Rg_2 input; V1_2 input
function y = fcn(u, Rf_2, R1_2, V2_2, Rg_2, V1_2)

y = ((((Rf_2+R1_2)*Rg_2*V2_2)/(u+Rg_2))-Rf_2*V1_2)/R1_2;

== matlab function simulink_10_04_procede/Boucle fermée /Écart consigne - ==
  data: Consigne input; y output; T_init input
function y = fcn(Consigne, T_init)

y = (-0.05*(Consigne-T_init))+Consigne;

== matlab function simulink_10_04_procede/Boucle fermée /Plaque/T0 2 R2 ==
  data: u input; y output; B2 input
function y = fcn(u, B2)
y = 10000*exp(B2*(1/(u+273.15) - 1/(298.15)));

== matlab function simulink_10_04_procede/Boucle fermée /Plaque/R1 2 V_op3 ==
  data: u input; y output; Rf_3 input; R1_3 input; V2_3 input; Rg_3 input; V1_3 input
function y = fcn_3(u, Rf_3, R1_3, V2_3, Rg_3, V1_3)

y = ((((Rf_3 + R1_3) * Rg_3 * V2_3) / (u + Rg_3)) - Rf_3 * V1_3) / R1_3;

== matlab function simulink_10_04_procede/Boucle fermée /Plaque/T0 2 R3 ==
  data: u input; y output; B3 input
function y = fcn(u, B3)
y = 10000*exp(B3*(1/(u+273.15) - 1/(298.15)));

== matlab function simulink_10_04_procede/Boucle fermée /V2 à T2/R2 2 T2 ==
  data: u input; y output; B2 input
function y = fcn(u, B2)
y = (1/((log(u/10000)/B2)+(1/(298.15))))-273.15;

== matlab function simulink_10_04_procede/Boucle fermée /V2 à T2/R1 2 V_op2 ==
  data: u input; y output; Rf_2 input; R1_2 input; V2_2 input; Rg_2 input; V1_2 input
function y = fcn(u, Rf_2, R1_2, V2_2, Rg_2, V1_2)

y = ((((Rf_2+R1_2)*Rg_2*V2_2)/(u+Rg_2))-Rf_2*V1_2)/R1_2;

== matlab function simulink_10_04_procede/Boucle fermée /V2 à T2/T0 2 R1 ==
  data: u input; y output; B1 input
function y = fcn(u, B1)
y = 10000*exp(B1*(1/(u+273.15) - 1/(298.15)));

== matlab function simulink_10_04_procede/Boucle ouverte/MATLAB Function ==
  data: u input; y output; T0 input
function y = fcn(u, T0)

if u > 0
    y = 0.0022*u^2 -0.0003 * T0^2 + 0.0002 * u * T0 + 0.2083 * u - 0.1342 * T0 + 3.2428;
    disp('puissance chaude');
else
    disp(u);
    y = 0.131449*u - 0.146920*T0 + 3.153989;
    disp(y);
    disp('puissance froide');


end

== matlab function simulink_10_04_procede/Boucle ouverte/Plaque/MATLAB Function ==
  data: u input; y output; R input
function y = fcn(u, R)

y = (u/R)^0.5;

== matlab function simulink_10_04_procede/Boucle fermée /Écart consigne + ==
  data: Consigne input; y output; T_init input
function y = fcn(Consigne, T_init)

y = (0.05*(Consigne-T_init))+Consigne;

== matlab function simulink_10_04_procede/Boucle ouverte/Plaque/MATLAB Function1 ==
  data: u input; y output; R input
function y = fcn(u, R)

y = (u/R)^0.5;

== matlab function simulink_10_04_procede/Boucle ouverte/Plaque/R1 2 T1 ==
  data: u input; y output; B1 input
function y = fcn(u, B1)
disp('B1');
disp(B1);
disp(u);
y = (1/((log(u/10000)/B1)+(1/(298.15))))-273.15;

== matlab function simulink_10_04_procede/Boucle ouverte/Plaque/R1 2 V_op1 ==
  data: u input; y output; Rf_1 input; R1_1 input; V2_1 input; Rg_1 input; V1_1 input
function y = fcn_1(u, Rf_1, R1_1, V2_1, Rg_1, V1_1)

y = ((((Rf_1 + R1_1) * Rg_1 * V2_1) / (u + Rg_1)) - Rf_1 * V1_1) / R1_1;

== matlab function simulink_10_04_procede/Boucle ouverte/Plaque/R1 2 V_op2 ==
  data: u input; y output; Rf_2 input; R1_2 input; V2_2 input; Rg_2 input; V1_2 input
function y = fcn(u, Rf_2, R1_2, V2_2, Rg_2, V1_2)

y = ((((Rf_2+R1_2)*Rg_2*V2_2)/(u+Rg_2))-Rf_2*V1_2)/R1_2;

== matlab function simulink_10_04_procede/Boucle ouverte/Plaque/R1 2 V_op3 ==
  data: u input; y output; Rf_3 input; R1_3 input; V2_3 input; Rg_3 input; V1_3 input
function y = fcn_3(u, Rf_3, R1_3, V2_3, Rg_3, V1_3)

y = ((((Rf_3 + R1_3) * Rg_3 * V2_3) / (u + Rg_3)) - Rf_3 * V1_3) / R1_3;

== matlab function simulink_10_04_procede/Boucle ouverte/Plaque/R2 2 T2 ==
  data: u input; y output; B2 input
function y = fcn(u, B2)
y = (1/((log(u/10000)/B2)+(1/(298.15))))-273.15;

== matlab function simulink_10_04_procede/Boucle ouverte/Plaque/R3 2 T3 ==
  data: u input; y output; B3 input
function y = fcn(u, B3)

y = (1/((log(u/10000)/B3)+(1/(298.15))))-273.15;

== matlab function simulink_10_04_procede/Boucle ouverte/Plaque/T0 2 R1 ==
  data: u input; y output; B1 input
function y = fcn(u, B1)
y = 10000*exp(B1*(1/(u+273.15) - 1/(298.15)));

== matlab function simulink_10_04_procede/Boucle ouverte/Plaque/T0 2 R2 ==
  data: u input; y output; B2 input
function y = fcn(u, B2)
y = 10000*exp(B2*(1/(u+273.15) - 1/(298.15)));

== matlab function simulink_10_04_procede/Boucle fermée /Plaque/MATLAB Function ==
  data: u input; y output; R input
function y = fcn(u, R)

y = (u/R)^0.5;

== matlab function simulink_10_04_procede/Boucle ouverte/Plaque/T0 2 R3 ==
  data: u input; y output; B3 input
function y = fcn(u, B3)
y = 10000*exp(B3*(1/(u+273.15) - 1/(298.15)));

== matlab function simulink_10_04_procede/Boucle ouverte/Plaque/V1 2 R1 ==
  data: u input; y output; Rf_1 input; Rg_1 input; R1_1 input; V2_1 input; V1_1 input
function y = fcn_1(u, Rf_1, Rg_1, R1_1, V2_1, V1_1)

% Calcul de la fraction
frac = ((Rf_1 + R1_1) * Rg_1 * V2_1) / (R1_1 * u + Rf_1 * V1_1);
disp(Rf_1);
disp(R1_1);
disp(V1_1);
disp(V2_1);
disp(u);

% Vérification : y doit rester positif
if frac - Rg_1 <= 0
    error('fcn_1 : tension u trop élevée, y devient négatif !');
end

% Calcul final
y = frac - Rg_1;

end

== matlab function simulink_10_04_procede/Boucle ouverte/Plaque/V2 2 R2 ==
  data: u input; y output; Rf_2 input; Rg_2 input; R1_2 input; V2_2 input; V1_2 input
function y = fcn_2(u, Rf_2, Rg_2, R1_2, V2_2, V1_2)

% Calcul de la fraction
frac = ((Rf_2 + R1_2) * Rg_2 * V2_2) / (R1_2 * u + Rf_2 * V1_2);

% Vérification : y doit rester positif
if frac - Rg_2 <= 0
    error('fcn_2 : tension u trop élevée, y devient négatif !');
end

% Calcul final
y = frac - Rg_2;

end

== matlab function simulink_10_04_procede/Boucle ouverte/Plaque/V3 2 R3 ==
  data: u input; y output; Rf_3 input; Rg_3 input; R1_3 input; V2_3 input; V1_3 input
function y = fcn_3(u, Rf_3, Rg_3, R1_3, V2_3, V1_3)

% Calcul de la fraction
frac = ((Rf_3 + R1_3) * Rg_3 * V2_3) / (R1_3 * u + Rf_3 * V1_3);

% Vérification : y doit rester positif
if frac - Rg_3 <= 0
    error('fcn_3 : tension u trop élevée, y devient négatif !');
end

% Calcul final
y = frac - Rg_3;

end

== matlab function simulink_10_04_procede/Boucle ouverte/V2 à T2/R1 2 V_op2 ==
  data: u input; y output; Rf_2 input; R1_2 input; V2_2 input; Rg_2 input; V1_2 input
function y = fcn(u, Rf_2, R1_2, V2_2, Rg_2, V1_2)

y = ((((Rf_2+R1_2)*Rg_2*V2_2)/(u+Rg_2))-Rf_2*V1_2)/R1_2;

== matlab function simulink_10_04_procede/Boucle ouverte/V2 à T2/R2 2 T2 ==
  data: u input; y output; B2 input
function y = fcn(u, B2)
y = (1/((log(u/10000)/B2)+(1/(298.15))))-273.15;

== matlab function simulink_10_04_procede/Boucle ouverte/V2 à T2/T0 2 R1 ==
  data: u input; y output; B1 input
function y = fcn(u, B1)
y = 10000*exp(B1*(1/(u+273.15) - 1/(298.15)));

== matlab function simulink_10_04_procede/Boucle ouverte/V2 à T2/V2 2 R2 ==
  data: u input; y output; Rf_2 input; Rg_2 input; R1_2 input; V2_2 input; V1_2 input
function y = fcn_2(u, Rf_2, Rg_2, R1_2, V2_2, V1_2)

% Calcul de la fraction
frac = ((Rf_2 + R1_2) * Rg_2 * V2_2) / (R1_2 * u + Rf_2 * V1_2);

% Vérification : y doit rester positif
if frac - Rg_2 <= 0
    error('fcn_2 : tension u trop élevée, y devient négatif !');
end

% Calcul final
y = frac - Rg_2;

end

== matlab function simulink_10_04_procede/Boucle fermée /MATLAB Function ==
  data: u input; y output; T0 input
function y = fcn(u, T0)

if u > 0
    y = 0.0022*u^2 -0.0003 * T0^2 + 0.0002 * u * T0 + 0.2083 * u - 0.1342 * T0 + 3.2428;
    disp('puissance chaude');
else
    disp(u);
    y = 0.131449*u - 0.146920*T0 + 3.153989;
    disp(y);
    disp('puissance froide');


end

== matlab function simulink_10_04_procede/Boucle ouverte/Écart consigne + ==
  data: Consigne input; y output; T_init input
function y = fcn(Consigne, T_init)

y = (0.05*(Consigne-T_init))+Consigne;

== matlab function simulink_10_04_procede/Boucle ouverte/Écart consigne - ==
  data: Consigne input; y output; T_init input
function y = fcn(Consigne, T_init)

y = (-0.05*(Consigne-T_init))+Consigne;

== matlab function simulink_10_04_procede/Boucle fermée /Plaque/MATLAB Function1 ==
  data: u input; y output; R input
function y = fcn(u, R)

y = (u/R)^0.5;

== matlab function simulink_10_04_procede/Boucle fermée /V2 à T2/V2 2 R2 ==
  data: u input; y output; Rf_2 input; Rg_2 input; R1_2 input; V2_2 input; V1_2 input
function y = fcn_2(u, Rf_2, Rg_2, R1_2, V2_2, V1_2)

% Calcul de la fraction
frac = ((Rf_2 + R1_2) * Rg_2 * V2_2) / (R1_2 * u + Rf_2 * V1_2);

% Vérification : y doit rester positif
if frac - Rg_2 <= 0
    error('fcn_2 : tension u trop élevée, y devient négatif !');
end

% Calcul final
y = frac - Rg_2;

end

== matlab function simulink_10_04_procede/Boucle fermée /Plaque/V2 2 R2 ==
  data: u input; y output; Rf_2 input; Rg_2 input; R1_2 input; V2_2 input; V1_2 input
function y = fcn_2(u, Rf_2, Rg_2, R1_2, V2_2, V1_2)

% Calcul de la fraction
frac = ((Rf_2 + R1_2) * Rg_2 * V2_2) / (R1_2 * u + Rf_2 * V1_2);

% Vérification : y doit rester positif
if frac - Rg_2 <= 0
    error('fcn_2 : tension u trop élevée, y devient négatif !');
end

% Calcul final
y = frac - Rg_2;

end

== matlab function simulink_10_04_procede/Boucle fermée /Plaque/V1 2 R1 ==
  data: u input; y output; Rf_1 input; Rg_1 input; R1_1 input; V2_1 input; V1_1 input
function y = fcn_1(u, Rf_1, Rg_1, R1_1, V2_1, V1_1)

% Calcul de la fraction
frac = ((Rf_1 + R1_1) * Rg_1 * V2_1) / (R1_1 * u + Rf_1 * V1_1);
disp(Rf_1);
disp(R1_1);
disp(V1_1);
disp(V2_1);
disp(u);

% Vérification : y doit rester positif
if frac - Rg_1 <= 0
    error('fcn_1 : tension u trop élevée, y devient négatif !');
end

% Calcul final
y = frac - Rg_1;

end

== matlab function simulink_10_04_procede/Boucle fermée /Plaque/V3 2 R3 ==
  data: u input; y output; Rf_3 input; Rg_3 input; R1_3 input; V2_3 input; V1_3 input
function y = fcn_3(u, Rf_3, Rg_3, R1_3, V2_3, V1_3)

% Calcul de la fraction
frac = ((Rf_3 + R1_3) * Rg_3 * V2_3) / (R1_3 * u + Rf_3 * V1_3);

% Vérification : y doit rester positif
if frac - Rg_3 <= 0
    error('fcn_3 : tension u trop élevée, y devient négatif !');
end

% Calcul final
y = frac - Rg_3;

end
